simulink model "model"  (R2015a)
settings: Solver=ode45  StartTime=0.0  StopTime=50  RelTol=1e-3
undefined symbols (not defined in the file): A, B, C, Ch, Kh, Ki, Kx, L, Lx, M, R
settings Model: Creator=jinkale  LastModifiedBy=jinkale

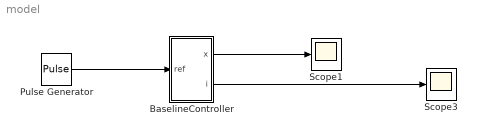
== system model ==
  BaselineController : Subsystem
  Pulse Generator : DiscretePulseGenerator  PulseType=Time based  Period=3  PulseWidth=50  PhaseDelay=10
  Scope1 : Scope
      settings: SaveName=ScopeData6
  Scope3 : Scope
      settings: SaveName=ScopeData3
  wires:
  Pulse Generator/1 -> BaselineController/1(ref)
  BaselineController/1(x) -> Scope1/1
  BaselineController/2(i) -> Scope3/1

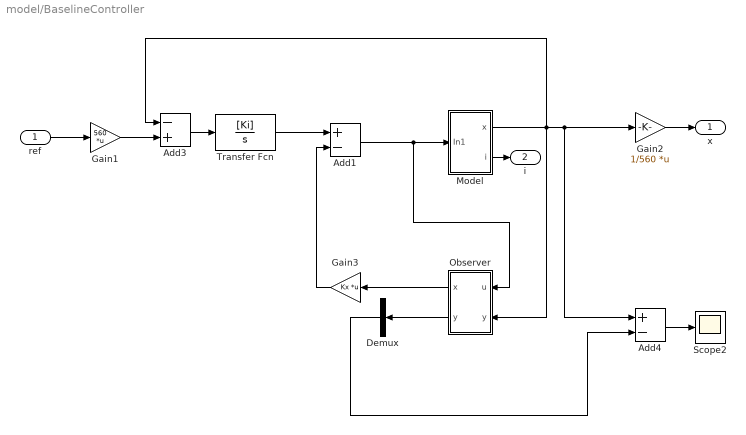
== system model/BaselineController ==
  ref : Inport
  Add1 : Sum  Inputs=+-
  Add3 : Sum  Inputs=-+
  Add4 : Sum  Inputs=+-
  Demux : Demux  Outputs=3
  Gain1 : Gain  Gain=560  Multiplication=Matrix(K*u) (u vector)
  Gain2 : Gain  Gain=1/560  Multiplication=Matrix(K*u) (u vector)
  Gain3 : Gain  Gain=Kx  Multiplication=Matrix(K*u)
  Model : Subsystem
  Observer : Subsystem
  Scope2 : Scope
      settings: SaveName=ScopeData5
  Transfer Fcn : TransferFcn  Numerator=[Ki]  Denominator=[1 0]
  x : Outport
  i : Outport  Port=2
  wires:
  Transfer Fcn/1 -> Add1/1
  Add3/1 -> Transfer Fcn/1
  Observer/2("y ") -> Demux/1
  Model/1(x) -> Observer/2(y), Add4/1, Gain2/1, Add3/1
  Add1/1 -> Observer/1(u), Model/1(In1)
  Demux/2 -> Add4/2
  Gain3/1 -> Add1/2
  Model/2(i) -> i/1
  ref/1 -> Gain1/1
  Observer/1("x ") -> Gain3/1
  Add4/1 -> Scope2/1
  Gain2/1 -> x/1
  Gain1/1 -> Add3/2

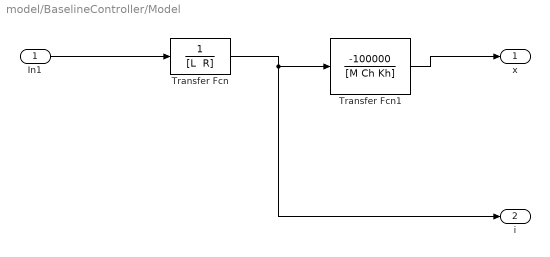
== system model/BaselineController/Model ==
  In1 : Inport
  Transfer Fcn : TransferFcn  Denominator="[L  R]"
  Transfer Fcn1 : TransferFcn  Numerator=[-100000]  Denominator=[M Ch Kh]
  x : Outport
  i : Outport  Port=2
  wires:
  Transfer Fcn/1 -> i/1, Transfer Fcn1/1
  In1/1 -> Transfer Fcn/1
  Transfer Fcn1/1 -> x/1

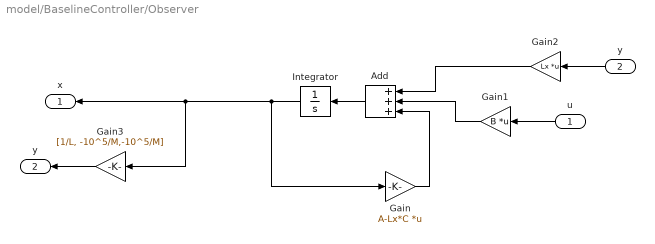
== system model/BaselineController/Observer ==
  u : Inport
  y : Inport  Port=2
  Add : Sum  Inputs=+++
  Gain : Gain  Gain=A-Lx*C  Multiplication=Matrix(K*u)
  Gain1 : Gain  Gain=B  Multiplication=Matrix(K*u)
  Gain2 : Gain  Gain=Lx  Multiplication=Matrix(K*u)
  Gain3 : Gain  Gain=[1/L, -10^5/M,-10^5/M]
  Integrator : Integrator
  "x " : Outport
  "y " : Outport  Port=2
  wires:
  Add/1 -> Integrator/1
  Integrator/1 -> Gain/1, Gain3/1, "x "/1
  Gain/1 -> Add/3
  Gain1/1 -> Add/2
  Gain2/1 -> Add/1
  y/1 -> Gain2/1
  u/1 -> Gain1/1
  Gain3/1 -> "y "/1
